simulink model "Simulator_template"  (Simulink 8.1)
settings: Solver=ode3  StartTime=0.0  StopTime=10  FixedStep=0.02  RelTol=1e-3
values from neighbouring files (symbols this model uses):
  g = 9.8065    [kostas_malakies.mat]    (also in kostas_malakies2.mat; load_PMModel.m = 9.81; main.m; main_last.m)
  la = l*sin(gamma+Theta)/J    [main.m]
  mass = 0.66    [kostas_malakies.mat]    (also in kostas_malakies2.mat; load_PMModel.m = 0.687; main_last.m)
  pitch = pitch/2/pi*180    [plotDataTest.m]
  Td_pitch_2ndOrd = 0.0464096828042    [kostas_malakies.mat]    (also in kostas_malakies2.mat)
  traj_FG =     [kostas.mat]    (also in kostas_malakies.mat; kostas_malakies2.mat; main_last.m = ReferenceCreator(maxdisty,maxdistz,scale_y,scale_z); traj_helix.mat)
  WallPos = 2.9    [kostas_malakies.mat]    (also in kostas_malakies2.mat; main_last.m)
  z = [-0.93079906702 -0.933865725994 -0.937557637691 -0.939011216164 -0.94143640995 -0.944628417492 -0.947235524654 -0.949601888657 -0.952827751637 -0.9567258358 -0.958320975304 -0.960991024971 ... (7988 elements, 7988x1)]    [kostas_malakies2.mat]    (also in plotDataTest.m = simout_data.signals.values(:,11))
undefined symbols (not defined in the file or in its folder): dynamics_pitch_2ndOrd
libraries: Hqaud_model_LIB_SI x4, Hquad_control_LIB_MPC x2
settings Model: Creator=andi  LastModifiedBy=root
settings DebuggingCC: InheritedTsInSrcMsg=none  StrictBusMsg=Warning
settings SFSimCC: SimParseCustomCode=off

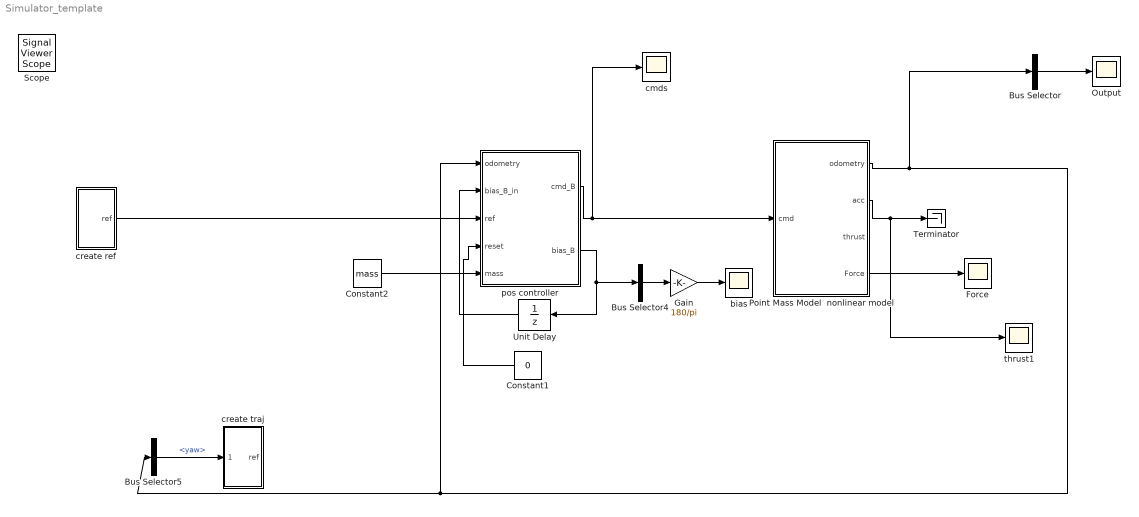
== system Simulator_template ==
  Bus Selector : BusSelector  OutputSignals=pos.x,vel.x_dot,rpy.pitch  OutputAsBus=on
  Bus Selector4 : BusSelector  OutputSignals=pitch_bias,roll_bias,thrust_bias  OutputAsBus=on
  Bus Selector5 : BusSelector  OutputSignals=rpy.yaw
  Constant1 : Constant  Value=0
  Constant2 : Constant  Value=mass
  Force : Scope
      settings: TimeRange=40  YMin=113.9130434782609  YMax=138.2608695652174  SaveName=ScopeData8
  Gain : Gain  Gain=180/pi
  Output : Scope
      settings: TimeRange=40  YMin=-0.5  YMax=0.5  SaveName=ScopeData4
  Point Mass Model  nonlinear model : Subsystem  AncestorBlock="Hqaud_model_LIB_SI/Point Mass Model  nonlinear model"
  Terminator : Terminator
  Unit Delay : UnitDelay  SampleTime=-1
  bias : Scope
      settings: TimeRange=39.996  YMin=-0.07  YMax=0.05
  cmds : Scope
      settings: TimeRange=40  YMin=-0.5  YMax=0.5
  create ref : Subsystem  AncestorBlock=Hquad_control_LIB_LQRI/create ref
  create traj : Subsystem
  pos controller : Subsystem  AncestorBlock=Hquad_control_LIB_MPC/pos controller
  thrust1 : Scope
      settings: TimeRange=40  YMin=-2  YMax=6  SaveName=ScopeData9
  Scope : SignalViewerScope  IOType=viewer  LegendLocations="321.25       180.625         123.5       128.125"  RefreshTime=0.035000
      settings: ShowLegends=on
  wires:
  Point Mass Model  nonlinear model/2(acc) -> Terminator/1, thrust1/1
  Constant1/1 -> pos controller/4(reset)
  Point Mass Model  nonlinear model/1(odometry) -> pos controller/1(odometry), Bus Selector5/1, Bus Selector/1
  pos controller/1(cmd_B) -> Point Mass Model  nonlinear model/1(cmd), cmds/1
  pos controller/2(bias_B) -> Unit Delay/1, Bus Selector4/1
  Bus Selector4/1 -> Gain/1
  Gain/1 -> bias/1
  Unit Delay/1 -> pos controller/2(bias_B_in)
  Constant2/1 -> pos controller/5(mass)
  Bus Selector5/1 -> create traj/1(yaw)  "<yaw>"
  create ref/1(ref) -> pos controller/3(ref)
  Point Mass Model  nonlinear model/4(Force) -> Force/1
  Bus Selector/1 -> Output/1

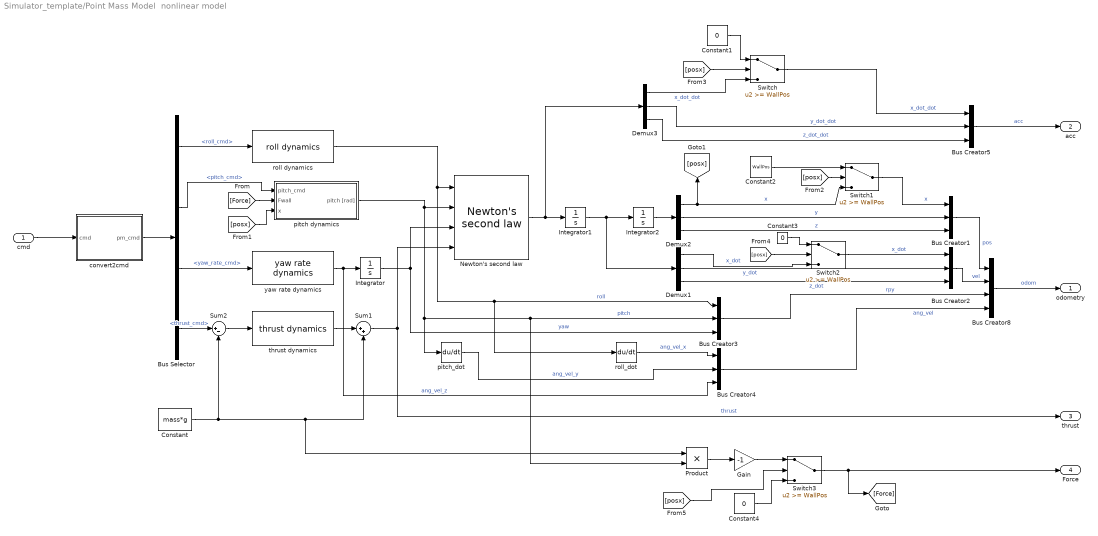
== system Simulator_template/Point Mass Model  nonlinear model ==
  cmd : Inport
  Bus Creator{1..5} (5 alike) : BusCreator  Inputs=3
  Bus Creator8 : BusCreator
  Bus Selector : BusSelector  OutputSignals=roll_cmd,pitch_cmd,yaw_rate_cmd,thrust_cmd
  Constant : Constant  Value=mass*g
  Constant1 : Constant  Value=0
  Constant2 : Constant  Value=WallPos
  Constant3 : Constant  Value=0
  Constant4 : Constant  Value=0
  Demux1 : Demux  Outputs=3
  Demux2 : Demux  Outputs=3
  Demux3 : Demux  Outputs=3
  Gain : Gain  Gain=-1
  Integrator : Integrator
  Integrator1 : Integrator
  Integrator2 : Integrator
  "Newton's second law  " : Hqaud_model_LIB_SI/Newton's second law  
  Product : Product
  Sum1 : Sum  Inputs=|++
  Sum2 : Sum  Inputs=|+-
  Switch{,1..3} (4 alike) : Switch  Threshold=WallPos
  convert2cmd : Subsystem
  "pitch dynamics  " : Subsystem  AncestorBlock=Hqaud_model_LIB_SI/pitch dynamics
  pitch_dot : Derivative
  roll dynamics : Hqaud_model_LIB_SI/roll dynamics
  roll_dot : Derivative
  "thrust dynamics  " : Hqaud_model_LIB_SI/thrust dynamics  
  "yaw rate dynamics  " : Hqaud_model_LIB_SI/yaw rate dynamics  
  odometry : Outport
  acc : Outport  Port=2
  "thrust   " : Outport  Port=3  PortDimensions=1
  Force : Outport  Port=4
  wires:
  convert2cmd/1(pm_cmd) -> Bus Selector/1
  Bus Selector/1 -> roll dynamics/1  "<roll_cmd>"
  "yaw rate dynamics  "/1 -> Integrator/1, Bus Creator4/3  "ang_vel_z"
  Integrator/1 -> "Newton's second law  "/3, Bus Creator3/3  "yaw"
  "thrust dynamics  "/1 -> Sum1/1
  "pitch dynamics  "/1("pitch [rad] ") -> "Newton's second law  "/2, Product/2, Bus Creator3/2, pitch_dot/1  "pitch"
  roll dynamics/1 -> "Newton's second law  "/1, Bus Creator3/1, roll_dot/1  "roll"
  "Newton's second law  "/1 -> Integrator1/1, Demux3/1
  Integrator1/1 -> Integrator2/1, Demux1/1
  Integrator2/1 -> Demux2/1
  Demux2/2 -> Bus Creator1/2  "y"
  Constant/1 -> Sum2/2, Product/1, Sum1/2
  cmd/1 -> convert2cmd/1(cmd)
  Bus Selector/2 -> "pitch dynamics  "/1("pitch_cmd  ")  "<pitch_cmd>"
  Bus Selector/3 -> "yaw rate dynamics  "/1  "<yaw_rate_cmd>"
  Bus Creator4/1 -> Bus Creator8/4  "ang_vel"
  Bus Creator3/1 -> Bus Creator8/3  "rpy"
  Bus Creator2/1 -> Bus Creator8/2  "vel"
  Bus Creator8/1 -> odometry/1  "odom"
  Demux2/3 -> Bus Creator1/3  "z"
  Demux2/1 -> Switch1/3, [posx]  "x"
  Demux1/2 -> Bus Creator2/2  "y_dot"
  Demux1/3 -> Bus Creator2/3  "z_dot"
  Bus Creator5/1 -> acc/1  "acc"
  Demux3/2 -> Bus Creator5/2  "y_dot_dot"
  Demux3/3 -> Bus Creator5/3  "z_dot_dot"
  Sum1/1 -> "Newton's second law  "/4, "thrust   "/1  "thrust"
  roll_dot/1 -> Bus Creator4/1  "ang_vel_x"
  pitch_dot/1 -> Bus Creator4/2  "ang_vel_y"
  Switch/1 -> Bus Creator5/1  "x_dot_dot"
  Bus Creator1/1 -> Bus Creator8/1  "pos"
  Constant1/1 -> Switch/1
  Demux3/1 -> Switch/3  "x_dot_dot"
  Constant2/1 -> Switch1/1
  Switch1/1 -> Bus Creator1/1  "x"
  Switch2/1 -> Bus Creator2/1  "x_dot"
  Constant3/1 -> Switch2/1
  Demux1/1 -> Switch2/3  "x_dot"
  Product/1 -> Gain/1
  [Force] -> "pitch dynamics  "/2(Fwall)
  [posx] -> "pitch dynamics  "/3(x)
  [posx] -> Switch1/2
  [posx] -> Switch/2
  [posx] -> Switch2/2
  Gain/1 -> Switch3/1
  Switch3/1 -> [Force], Force/1
  Constant4/1 -> Switch3/3
  [posx] -> Switch3/2
  Bus Selector/4 -> Sum2/1  "<thrust_cmd>"
  Sum2/1 -> "thrust dynamics  "/1

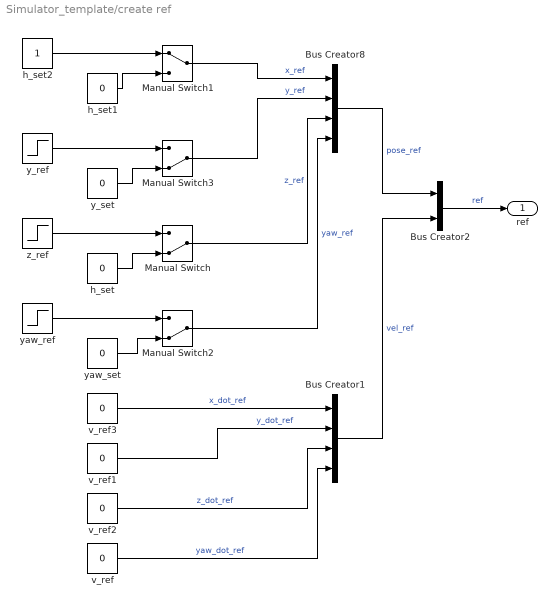
== system Simulator_template/create ref ==
  Bus Creator1 : BusCreator
  Bus Creator2 : BusCreator  Inputs=2
  Bus Creator8 : BusCreator
  Manual Switch : ManualSwitch  CurrentSetting=0
  Manual Switch1 : ManualSwitch
  Manual Switch2 : ManualSwitch  CurrentSetting=0
  Manual Switch3 : ManualSwitch  CurrentSetting=0
  h_set : Constant  Value=0  OutDataTypeStr=double  SampleTime=-1
  h_set1 : Constant  Value=0  OutDataTypeStr=double  SampleTime=-1
  h_set2 : Constant  OutDataTypeStr=double  SampleTime=-1
  v_ref{,1..3} (4 alike) : Constant  Value=0  OutDataTypeStr=double  SampleTime=-1
  y_ref : Step  Time=15  SampleTime=0
  y_set : Constant  Value=0  OutDataTypeStr=double  SampleTime=-1
  yaw_ref : Step  Time=20  After=pi  SampleTime=0
  "yaw_set  " : Constant  Value=0  OutDataTypeStr=double  SampleTime=-1
  z_ref : Step  Time=15  SampleTime=0
  ref : Outport
  wires:
  h_set2/1 -> Manual Switch1/1
  v_ref2/1 -> Bus Creator1/3  "z_dot_ref"
  v_ref1/1 -> Bus Creator1/2  "y_dot_ref"
  v_ref3/1 -> Bus Creator1/1  "x_dot_ref"
  v_ref/1 -> Bus Creator1/4  "yaw_dot_ref"
  Manual Switch/1 -> Bus Creator8/3  "z_ref"
  Manual Switch2/1 -> Bus Creator8/4  "yaw_ref"
  Manual Switch3/1 -> Bus Creator8/2  "y_ref"
  Manual Switch1/1 -> Bus Creator8/1  "x_ref"
  Bus Creator1/1 -> Bus Creator2/2  "vel_ref"
  Bus Creator8/1 -> Bus Creator2/1  "pose_ref"
  Bus Creator2/1 -> ref/1  "ref"
  h_set1/1 -> Manual Switch1/2
  y_set/1 -> Manual Switch3/2
  y_ref/1 -> Manual Switch3/1
  z_ref/1 -> Manual Switch/1
  h_set/1 -> Manual Switch/2
  "yaw_set  "/1 -> Manual Switch2/2
  yaw_ref/1 -> Manual Switch2/1

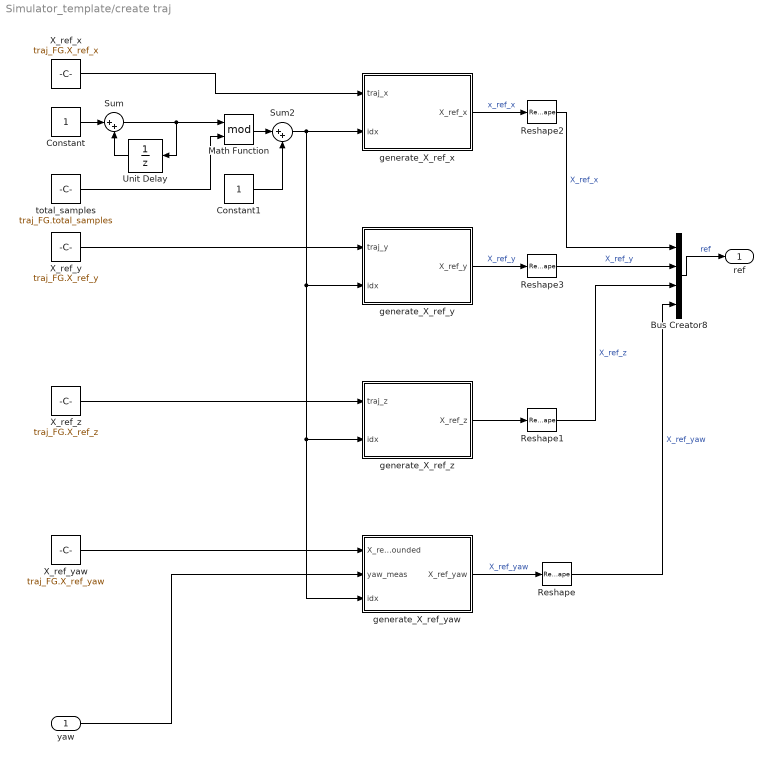
== system Simulator_template/create traj ==
  yaw : Inport
  Bus Creator8 : BusCreator
  Constant : Constant
  Constant1 : Constant
  Math Function : Math  Operator=mod  SaturateOnIntegerOverflow=on
  Reshape{,1..3} (4 alike) : Reshape
  Sum : Sum  Inputs=|++
  Sum2 : Sum  Inputs=|++
  Unit Delay : UnitDelay  SampleTime=-1
  X_ref_x : Constant  Value=traj_FG.X_ref_x
  X_ref_y : Constant  Value=traj_FG.X_ref_y
  X_ref_yaw : Constant  Value=traj_FG.X_ref_yaw
  X_ref_z : Constant  Value=traj_FG.X_ref_z
  generate_X_ref_x : MATLAB Function  TreatAsAtomicUnit=on
  generate_X_ref_y : MATLAB Function  TreatAsAtomicUnit=on
  generate_X_ref_yaw : MATLAB Function  TreatAsAtomicUnit=on
  generate_X_ref_z : MATLAB Function  TreatAsAtomicUnit=on
  total_samples : Constant  Value=traj_FG.total_samples
  ref : Outport
  wires:
  Bus Creator8/1 -> ref/1  "ref"
  Constant/1 -> Sum/1
  Unit Delay/1 -> Sum/2
  Sum/1 -> Unit Delay/1, Math Function/1
  total_samples/1 -> Math Function/2
  Math Function/1 -> Sum2/1
  X_ref_yaw/1 -> generate_X_ref_yaw/1(X_ref_yaw_unbounded)
  Constant1/1 -> Sum2/2
  yaw/1 -> generate_X_ref_yaw/2(yaw_meas)
  Sum2/1 -> generate_X_ref_x/2(idx), generate_X_ref_yaw/3(idx), generate_X_ref_z/2(idx), generate_X_ref_y/2(idx)
  Reshape/1 -> Bus Creator8/4  "X_ref_yaw"
  generate_X_ref_yaw/1(X_ref_yaw) -> Reshape/1  "X_ref_yaw"
  generate_X_ref_z/1(X_ref_z) -> Reshape1/1
  Reshape1/1 -> Bus Creator8/3  "X_ref_z"
  X_ref_z/1 -> generate_X_ref_z/1(traj_z)
  X_ref_y/1 -> generate_X_ref_y/1(traj_y)
  X_ref_x/1 -> generate_X_ref_x/1(traj_x)
  generate_X_ref_x/1(X_ref_x) -> Reshape2/1  "x_ref_x"
  generate_X_ref_y/1(X_ref_y) -> Reshape3/1  "X_ref_y"
  Reshape2/1 -> Bus Creator8/1  "X_ref_x"
  Reshape3/1 -> Bus Creator8/2  "X_ref_y"

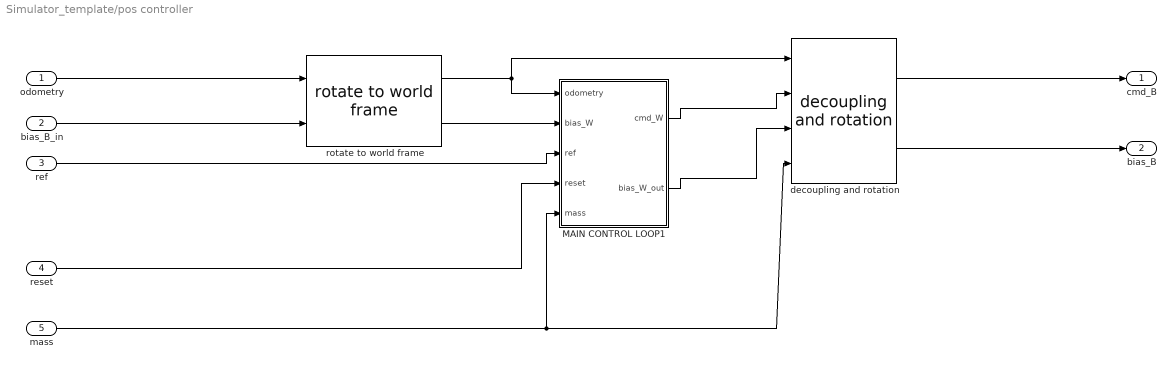
== system Simulator_template/pos controller ==
  odometry : Inport
  bias_B_in : Inport  Port=2
  ref : Inport  Port=3
  reset : Inport  Port=4
  mass : Inport  Port=5
  MAIN CONTROL LOOP1 : Subsystem  Priority=2  AncestorBlock=Hquad_control_LIB_MPC/MAIN CONTROL LOOP  TreatAsAtomicUnit=on
  decoupling and rotation : Hquad_control_LIB_MPC/decoupling and rotation  Priority=3
  rotate to world frame : Hquad_control_LIB_MPC/rotate to world frame  Priority=1
  cmd_B : Outport
  bias_B : Outport  Port=2
  wires:
  mass/1 -> decoupling and rotation/4, MAIN CONTROL LOOP1/5(mass)
  bias_B_in/1 -> rotate to world frame/2
  rotate to world frame/2 -> MAIN CONTROL LOOP1/2(bias_W)
  decoupling and rotation/2 -> bias_B/1
  decoupling and rotation/1 -> cmd_B/1
  MAIN CONTROL LOOP1/2(bias_W_out) -> decoupling and rotation/3
  rotate to world frame/1 -> decoupling and rotation/1, MAIN CONTROL LOOP1/1(odometry)
  ref/1 -> MAIN CONTROL LOOP1/3(ref)
  reset/1 -> MAIN CONTROL LOOP1/4(reset)
  MAIN CONTROL LOOP1/1(cmd_W) -> decoupling and rotation/2
  odometry/1 -> rotate to world frame/1

== system Simulator_template/Point Mass Model  nonlinear model/convert2cmd ==
  cmd : Inport
  Bus Creator8 : BusCreator
  Bus Selector : BusSelector  OutputSignals=pitch_cmd,roll_cmd,thrust_cmd,yaw_rate_cmd
  pm_cmd : Outport
  wires:
  Bus Selector/3 -> Bus Creator8/3  "<thrust_cmd>"
  Bus Selector/4 -> Bus Creator8/4  "<yaw_rate_cmd>"
  Bus Selector/2 -> Bus Creator8/2  "<roll_cmd>"
  Bus Selector/1 -> Bus Creator8/1  "<pitch_cmd>"
  cmd/1 -> Bus Selector/1
  Bus Creator8/1 -> pm_cmd/1

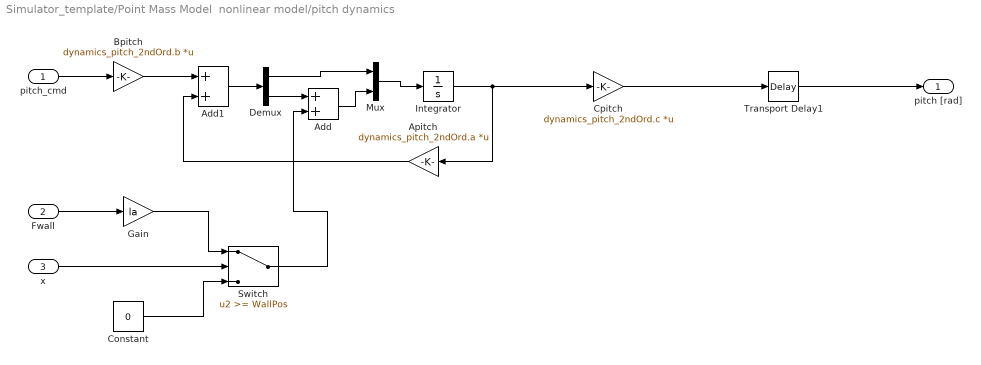
== system Simulator_template/Point Mass Model  nonlinear model/pitch dynamics   ==
  "pitch_cmd  " : Inport  PortDimensions=1
  Fwall : Inport  Port=2
  x : Inport  Port=3
  Add : Sum
  Add1 : Sum
  Apitch : Gain  Gain=dynamics_pitch_2ndOrd.a  Multiplication=Matrix(K*u)
  Bpitch : Gain  Gain=dynamics_pitch_2ndOrd.b  Multiplication=Matrix(K*u)
  Constant : Constant  Value=0
  Cpitch : Gain  Gain=dynamics_pitch_2ndOrd.c  Multiplication=Matrix(K*u)
  Demux : Demux  Outputs=2
  Gain : Gain  Gain=la
  Integrator : Integrator
  Mux : Mux  Inputs=2
  Switch : Switch  Threshold=WallPos
  Transport Delay1 : TransportDelay  DelayTime=Td_pitch_2ndOrd  PadeOrder=delay_pade_order
  "pitch [rad] " : Outport  PortDimensions=1
  wires:
  Demux/2 -> Add/1
  x/1 -> Switch/2
  Switch/1 -> Add/2
  Fwall/1 -> Gain/1
  Gain/1 -> Switch/1
  Constant/1 -> Switch/3
  Integrator/1 -> Cpitch/1, Apitch/1
  Apitch/1 -> Add1/2
  "pitch_cmd  "/1 -> Bpitch/1
  Bpitch/1 -> Add1/1
  Transport Delay1/1 -> "pitch [rad] "/1
  Cpitch/1 -> Transport Delay1/1
  Add1/1 -> Demux/1
  Add/1 -> Mux/2
  Demux/1 -> Mux/1
  Mux/1 -> Integrator/1

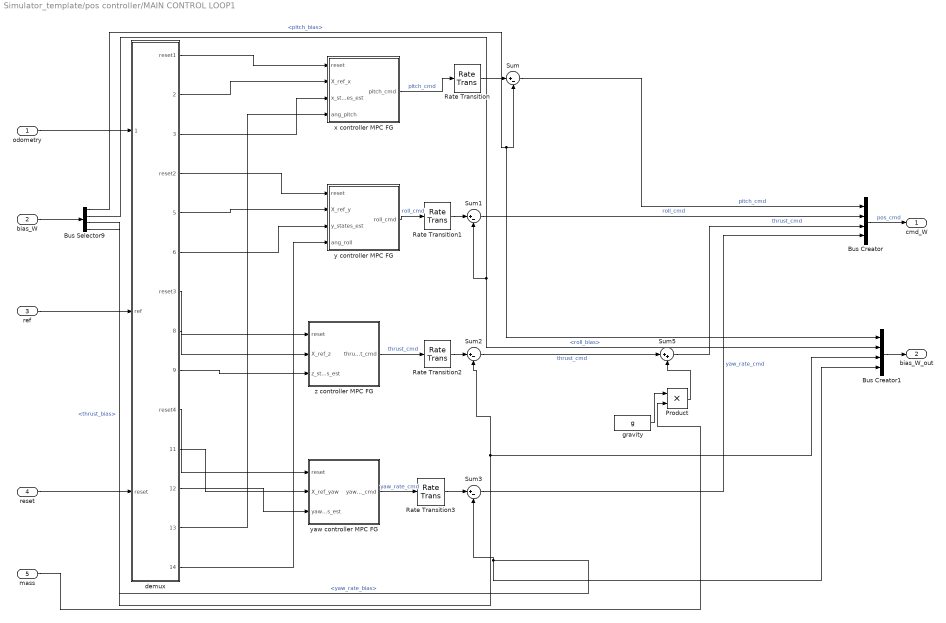
== system Simulator_template/pos controller/MAIN CONTROL LOOP1 ==
  odometry : Inport
  bias_W : Inport  Port=2
  ref : Inport  Port=3
  reset : Inport  Port=4
  mass : Inport  Port=5
  Bus Creator : BusCreator
  Bus Creator1 : BusCreator
  Bus Selector9 : BusSelector  OutputSignals=pitch_bias,roll_bias,thrust_bias,yaw_rate_bias
  Product : Product  RndMeth=Zero
  Rate Transition{,1..3} (4 alike) : RateTransition
  Sum{,1..3} (4 alike) : Sum  Inputs=|+-
  Sum5 : Sum  Inputs=|++
  demux : Subsystem
  gravity : Constant  Value=g
  "x controller MPC FG  " : Subsystem  AncestorBlock=Hquad_control_LIB_MPC/x controller MPC FG
  y controller MPC FG : Subsystem  AncestorBlock=Hquad_control_LIB_MPC/y controller MPC FG
  yaw controller MPC FG : Subsystem  AncestorBlock=Hquad_control_LIB_MPC/yaw controller MPC FG
  z controller MPC FG : Subsystem  AncestorBlock=Hquad_control_LIB_MPC/z controller MPC FG
  cmd_W : Outport
  bias_W_out : Outport  Port=2
  wires:
  Bus Selector9/4 -> Sum3/2, Bus Creator1/4  "<yaw_rate_bias>"
  Sum3/1 -> Bus Creator/4  "yaw_rate_cmd"
  yaw controller MPC FG/1(yaw_rate_cmd) -> Rate Transition3/1  "yaw_rate_cmd"
  Bus Selector9/3 -> Sum2/2, Bus Creator1/3  "<thrust_bias>"
  Bus Selector9/1 -> Sum/2, Bus Creator1/1  "<pitch_bias>"
  demux/12(yaw_states_meas) -> yaw controller MPC FG/3("yaw_states_est  ")
  Bus Selector9/2 -> Bus Creator1/2, Sum1/2  "<roll_bias>"
  bias_W/1 -> Bus Selector9/1
  Sum5/1 -> Bus Creator/3  "thrust_cmd"
  Bus Creator1/1 -> bias_W_out/1
  Sum2/1 -> Sum5/1  "thrust_cmd"
  z controller MPC FG/1(thrust_cmd) -> Rate Transition2/1  "thrust_cmd"
  Sum1/1 -> Bus Creator/2  "roll_cmd"
  y controller MPC FG/1(roll_cmd) -> Rate Transition1/1  "roll_cmd"
  Sum/1 -> Bus Creator/1  "pitch_cmd"
  "x controller MPC FG  "/1("pitch_cmd   ") -> Rate Transition/1  "pitch_cmd"
  demux/8(X_ref_z) -> z controller MPC FG/2(X_ref_z)
  demux/2(X_ref_x) -> "x controller MPC FG  "/2("X_ref_x  ")
  odometry/1 -> demux/1(odometry)
  ref/1 -> demux/2(ref)
  reset/1 -> demux/3(reset)
  demux/1(reset1) -> "x controller MPC FG  "/1(reset)
  demux/4(reset2) -> y controller MPC FG/1(reset)
  demux/5(X_ref_y) -> y controller MPC FG/2("X_ref_y  ")
  demux/7(reset3) -> z controller MPC FG/1(reset)
  demux/10(reset4) -> yaw controller MPC FG/1(reset)
  Bus Creator/1 -> cmd_W/1  "pos_cmd"
  demux/11(X_ref_yaw) -> yaw controller MPC FG/2(X_ref_yaw)
  mass/1 -> Product/2
  Product/1 -> Sum5/2
  gravity/1 -> Product/1
  demux/3(x_states_meas) -> "x controller MPC FG  "/3("x_states_est  ")
  demux/6(y_states_meas) -> y controller MPC FG/3("y_states_est  ")
  demux/9(z_states_meas) -> z controller MPC FG/3("z_states_est  ")
  demux/13(ang_pitch) -> "x controller MPC FG  "/4(ang_pitch)
  demux/14(ang_roll) -> y controller MPC FG/4(ang_roll)
  Rate Transition/1 -> Sum/1
  Rate Transition1/1 -> Sum1/1
  Rate Transition2/1 -> Sum2/1
  Rate Transition3/1 -> Sum3/1

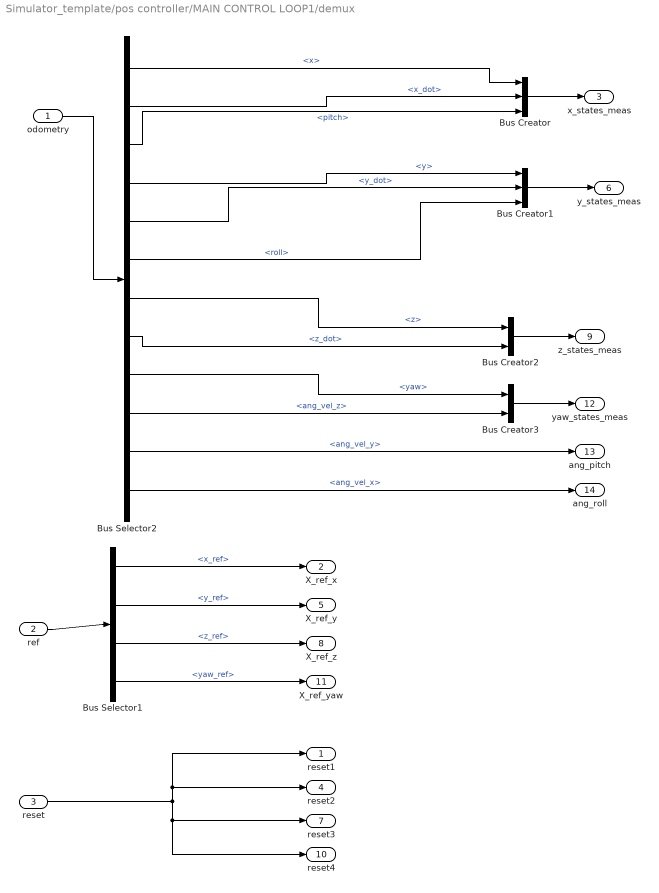
== system Simulator_template/pos controller/MAIN CONTROL LOOP1/demux ==
  odometry : Inport
  ref : Inport  Port=2
  reset : Inport  Port=3
  Bus Creator : BusCreator  Inputs=3
  Bus Creator1 : BusCreator  Inputs=3
  Bus Creator2 : BusCreator  Inputs=2
  Bus Creator3 : BusCreator  Inputs=2
  Bus Selector1 : BusSelector  OutputSignals=pose_ref.x_ref,pose_ref.y_ref,pose_ref.z_ref,pose_ref.yaw_ref
  Bus Selector2 : BusSelector  OutputSignals=pos.x,vel.x_dot,rpy.pitch,pos.y,vel.y_dot,rpy.roll,pos.z,vel.z_dot,rpy.yaw,ang_vel.ang_vel_z,ang_vel.ang_vel_y,ang_vel.ang_vel_x
  reset1 : Outport
  X_ref_x : Outport  Port=2
  x_states_meas : Outport  Port=3  PortDimensions=3
  reset2 : Outport  Port=4
  X_ref_y : Outport  Port=5
  y_states_meas : Outport  Port=6  PortDimensions=3
  reset3 : Outport  Port=7
  X_ref_z : Outport  Port=8
  z_states_meas : Outport  Port=9  PortDimensions=2
  reset4 : Outport  Port=10
  X_ref_yaw : Outport  Port=11
  yaw_states_meas : Outport  Port=12  PortDimensions=2
  ang_pitch : Outport  Port=13
  ang_roll : Outport  Port=14
  wires:
  Bus Selector1/4 -> X_ref_yaw/1  "<yaw_ref>"
  Bus Selector1/3 -> X_ref_z/1  "<z_ref>"
  Bus Selector2/3 -> Bus Creator/3  "<pitch>"
  odometry/1 -> Bus Selector2/1
  Bus Creator/1 -> x_states_meas/1
  Bus Selector2/1 -> Bus Creator/1  "<x>"
  Bus Selector2/2 -> Bus Creator/2  "<x_dot>"
  Bus Selector2/5 -> Bus Creator1/2  "<y_dot>"
  Bus Selector2/7 -> Bus Creator2/1  "<z>"
  Bus Selector2/8 -> Bus Creator2/2  "<z_dot>"
  Bus Selector2/9 -> Bus Creator3/1  "<yaw>"
  Bus Selector2/10 -> Bus Creator3/2  "<ang_vel_z>"
  Bus Creator2/1 -> z_states_meas/1
  Bus Creator3/1 -> yaw_states_meas/1
  ref/1 -> Bus Selector1/1
  Bus Selector1/1 -> X_ref_x/1  "<x_ref>"
  Bus Selector1/2 -> X_ref_y/1  "<y_ref>"
  reset/1 -> reset3/1, reset4/1, reset2/1, reset1/1
  Bus Selector2/6 -> Bus Creator1/3  "<roll>"
  Bus Selector2/4 -> Bus Creator1/1  "<y>"
  Bus Creator1/1 -> y_states_meas/1
  Bus Selector2/11 -> ang_pitch/1  "<ang_vel_y>"
  Bus Selector2/12 -> ang_roll/1  "<ang_vel_x>"

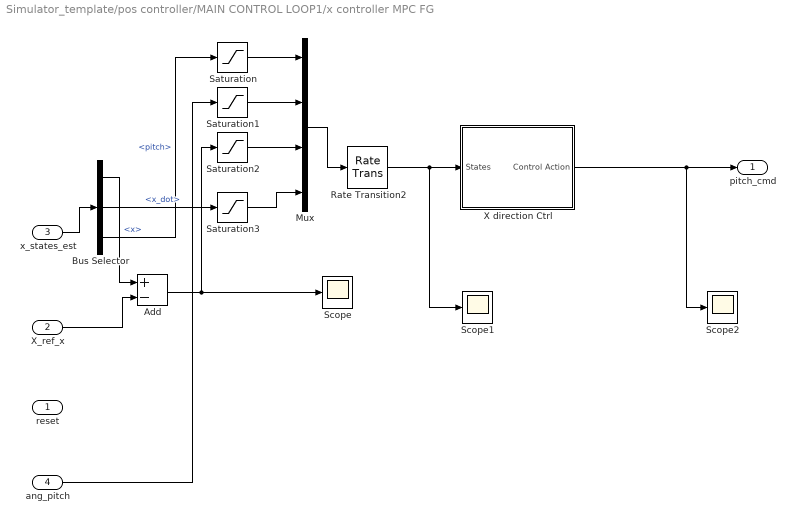
== system Simulator_template/pos controller/MAIN CONTROL LOOP1/x controller MPC FG   ==
  reset : Inport  PortDimensions=1
  "X_ref_x  " : Inport  Port=2
  "x_states_est  " : Inport  Port=3
  ang_pitch : Inport  Port=4  PortDimensions=1
  Add : Sum  Inputs=+-
  Bus Selector : BusSelector  OutputSignals=x,x_dot,pitch
  Mux : Mux
  Rate Transition2 : RateTransition
  Saturation : Saturate  UpperLimit=0.2094  LowerLimit=-0.2094
  Saturation1 : Saturate  UpperLimit=2  LowerLimit=-2
  Saturation2 : Saturate  UpperLimit=0  LowerLimit=-1
  Saturation3 : Saturate  UpperLimit=1  LowerLimit=-1
  Scope : Scope
      settings: SaveName=ScopeData2
  Scope1 : Scope
      settings: SaveName=ScopeData3
  Scope2 : Scope
      settings: SaveName=ScopeData5
  X direction Ctrl : Subsystem  AncestorBlock=mpt_sim/Explicit Controller  mask(MPT Controller){}
      mask help: Evaluates explicit controller for a given state.
      mask Help: Evaluation of an explicit control law is performed by the C-code S-function "mpt_getInput_sfunc", which requires the controller to be exported to C-code using "exportToC".
      mask Display: image(imread('mpt_ctrl.jpg'));
  "pitch_cmd   " : Outport  PortDimensions=1
  wires:
  "X_ref_x  "/1 -> Add/2
  "x_states_est  "/1 -> Bus Selector/1
  Add/1 -> Scope/1, Saturation2/1
  X direction Ctrl/1(Control Action) -> Scope2/1, "pitch_cmd   "/1
  Mux/1 -> Rate Transition2/1
  ang_pitch/1 -> Saturation1/1
  Bus Selector/1 -> Add/1  "<x>"
  Bus Selector/2 -> Saturation3/1  "<x_dot>"
  Bus Selector/3 -> Saturation/1  "<pitch>"
  Rate Transition2/1 -> Scope1/1, X direction Ctrl/1(States)
  Saturation/1 -> Mux/1
  Saturation1/1 -> Mux/2
  Saturation2/1 -> Mux/3
  Saturation3/1 -> Mux/4

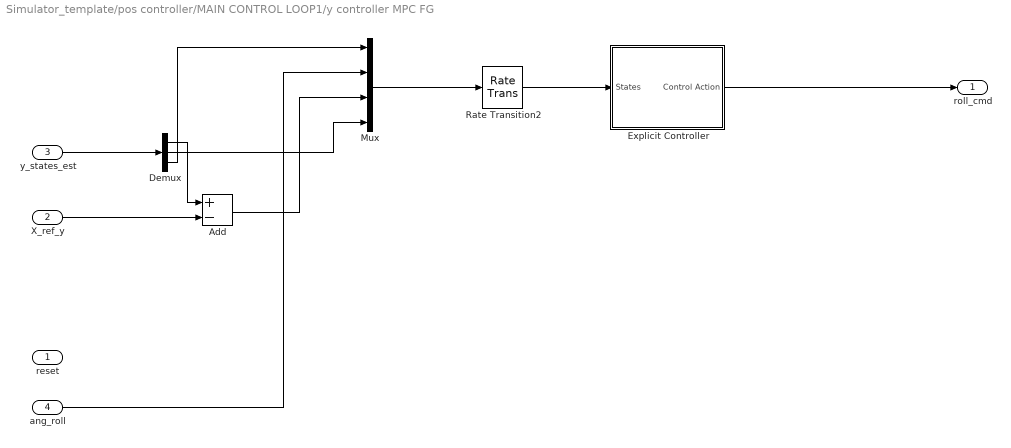
== system Simulator_template/pos controller/MAIN CONTROL LOOP1/y controller MPC FG ==
  reset : Inport  PortDimensions=1
  "X_ref_y  " : Inport  Port=2
  "y_states_est  " : Inport  Port=3
  ang_roll : Inport  Port=4  PortDimensions=1
  Add : Sum  Inputs=+-
  Demux : Demux  Outputs=3
  Explicit Controller : Subsystem  AncestorBlock=mpt_sim/Explicit Controller  mask(MPT Controller){}
      mask help: Evaluates explicit controller for a given state.
      mask Help: Evaluation of an explicit control law is performed by the C-code S-function "mpt_getInput_sfunc", which requires the controller to be exported to C-code using "exportToC".
      mask Display: image(imread('mpt_ctrl.jpg'));
  Mux : Mux
  Rate Transition2 : RateTransition
  roll_cmd : Outport  PortDimensions=1
  wires:
  "X_ref_y  "/1 -> Add/2
  "y_states_est  "/1 -> Demux/1
  Demux/1 -> Add/1
  Mux/1 -> Rate Transition2/1
  Explicit Controller/1(Control Action) -> roll_cmd/1
  Add/1 -> Mux/3
  Demux/2 -> Mux/4
  Demux/3 -> Mux/1
  ang_roll/1 -> Mux/2
  Rate Transition2/1 -> Explicit Controller/1(States)

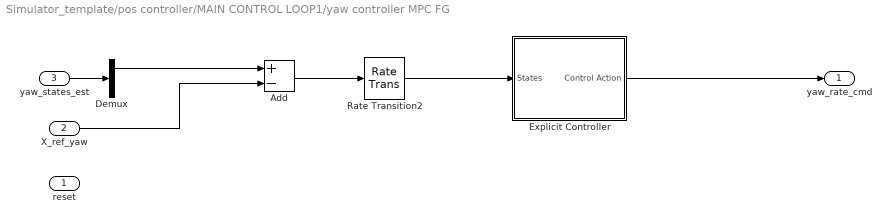
== system Simulator_template/pos controller/MAIN CONTROL LOOP1/yaw controller MPC FG ==
  reset : Inport  PortDimensions=1
  X_ref_yaw : Inport  Port=2
  "yaw_states_est  " : Inport  Port=3
  Add : Sum  Inputs=+-
  Demux : Demux  Outputs=2
  Explicit Controller : Subsystem  AncestorBlock=mpt_sim/Explicit Controller  mask(MPT Controller){}
      mask help: Evaluates explicit controller for a given state.
      mask Help: Evaluation of an explicit control law is performed by the C-code S-function "mpt_getInput_sfunc", which requires the controller to be exported to C-code using "exportToC".
      mask Display: image(imread('mpt_ctrl.jpg'));
  Rate Transition2 : RateTransition
  yaw_rate_cmd : Outport  PortDimensions=1
  wires:
  X_ref_yaw/1 -> Add/2
  "yaw_states_est  "/1 -> Demux/1
  Demux/1 -> Add/1
  Add/1 -> Rate Transition2/1
  Explicit Controller/1(Control Action) -> yaw_rate_cmd/1
  Rate Transition2/1 -> Explicit Controller/1(States)

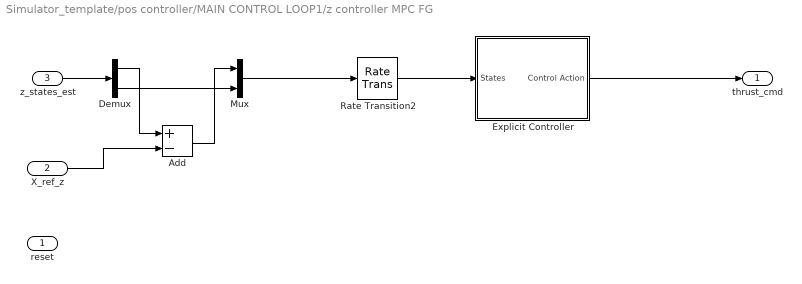
== system Simulator_template/pos controller/MAIN CONTROL LOOP1/z controller MPC FG ==
  reset : Inport  PortDimensions=1
  X_ref_z : Inport  Port=2
  "z_states_est  " : Inport  Port=3
  Add : Sum  Inputs=+-
  Demux : Demux  Outputs=2
  Explicit Controller : Subsystem  AncestorBlock=mpt_sim/Explicit Controller  mask(MPT Controller){}
      mask help: Evaluates explicit controller for a given state.
      mask Help: Evaluation of an explicit control law is performed by the C-code S-function "mpt_getInput_sfunc", which requires the controller to be exported to C-code using "exportToC".
      mask Display: image(imread('mpt_ctrl.jpg'));
  Mux : Mux  Inputs=2
  Rate Transition2 : RateTransition
  thrust_cmd : Outport  PortDimensions=1
  wires:
  "z_states_est  "/1 -> Demux/1
  Demux/2 -> Mux/2
  Demux/1 -> Add/1
  X_ref_z/1 -> Add/2
  Add/1 -> Mux/1
  Mux/1 -> Rate Transition2/1
  Explicit Controller/1(Control Action) -> thrust_cmd/1
  Rate Transition2/1 -> Explicit Controller/1(States)

== system Simulator_template/pos controller/MAIN CONTROL LOOP1/x controller MPC FG  /X direction Ctrl ==
  States : Inport
  S-Function : S-Function  FunctionName=mpt_getInput_sfunc_Xdirection  EnableBusSupport=off
  Control Action : Outport
  wires:
  S-Function/1 -> Control Action/1
  States/1 -> S-Function/1

== system Simulator_template/pos controller/MAIN CONTROL LOOP1/y controller MPC FG/Explicit Controller ==
  States : Inport
  S-Function : S-Function  FunctionName=mpt_getInput_sfunc_Ydirection  EnableBusSupport=off
  Control Action : Outport
  wires:
  S-Function/1 -> Control Action/1
  States/1 -> S-Function/1

== system Simulator_template/pos controller/MAIN CONTROL LOOP1/yaw controller MPC FG/Explicit Controller ==
  States : Inport
  S-Function : S-Function  FunctionName=mpt_getInput_sfunc_YawCtrl  EnableBusSupport=off
  Control Action : Outport
  wires:
  S-Function/1 -> Control Action/1
  States/1 -> S-Function/1

== system Simulator_template/pos controller/MAIN CONTROL LOOP1/z controller MPC FG/Explicit Controller ==
  States : Inport
  S-Function : S-Function  FunctionName=mpt_getInput_sfunc_Zdirection  EnableBusSupport=off
  Control Action : Outport
  wires:
  S-Function/1 -> Control Action/1
  States/1 -> S-Function/1

== matlab function create traj/generate_X_ref_z ==
  data: traj_z input double; X_ref_z output double; idx input double
function X_ref_z  = fcn(traj_z,idx)

pred_horizon_z=30;

X_ref_z=traj_z(:,idx:idx+pred_horizon_z);

== matlab function create traj/generate_X_ref_y ==
  data: traj_y input double; X_ref_y output double; idx input double
function X_ref_y  = fcn(traj_y,idx)

pred_horizon_y=30;

X_ref_y=traj_y(:,idx:idx+pred_horizon_y);

== matlab function create traj/generate_X_ref_x ==
  data: traj_x input double; X_ref_x output double; idx input double
function X_ref_x  = fcn(traj_x,idx)

pred_horizon_x=30;

X_ref_x=traj_x(:,idx:idx+pred_horizon_x);

== matlab function create traj/generate_X_ref_yaw ==
  data: X_ref_yaw_unbounded input double; X_ref_yaw output double; yaw_meas input double; idx input double
function X_ref_yaw  = fcn(X_ref_yaw_unbounded,yaw_meas,idx)

pred_horizon_yaw=30;

yaw0=X_ref_yaw_unbounded(1,idx);
yaw_diff=yaw_meas-yaw0;


yaw_offset=round(yaw_diff/(2*pi))*2*pi;

X_ref_yaw=[X_ref_yaw_unbounded(1,idx:idx+pred_horizon_yaw)+yaw_offset;...
    X_ref_yaw_unbounded(2,idx:idx+pred_horizon_yaw)];
